simulink subsystem "rss_ECUCircuitry"  (R2024a)
settings: Solver=VariableStepAuto  StartTime=0.0  StopTime=10.0  RelTol=1e-3
libraries: fl_lib x41, nesl_utility x19, ee_lib x1
settings Model: Creator=pav2ofo  LastModifiedBy=pav2ofo

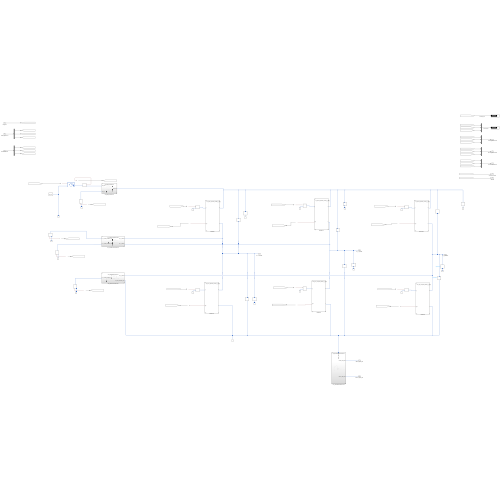
[thumbnail: Simulink's stored preview of the top-level diagram]
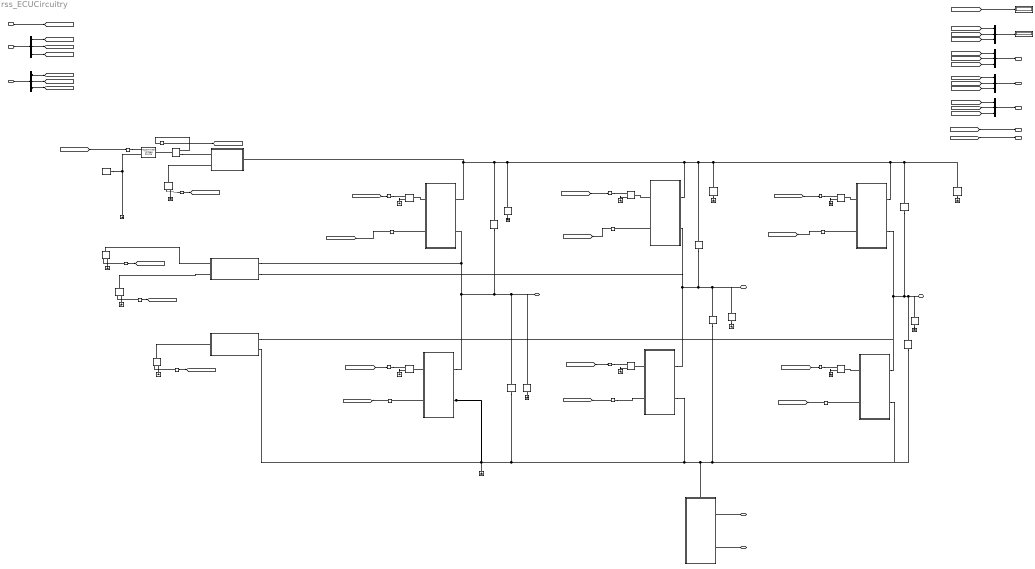
== system rss_ECUCircuitry ==
  vtSplyVolt : Inport
  iXYZHighGateCurr : Inport  Port=2
  iXYZLowGateCurr : Inport  Port=3
  Capacitor1 : fl_lib/Electrical/Electrical Elements/Capacitor  c=cstDrnPhsCpct F  r=cstDrnPhsCpcrRstn Ohm  g=0 1/Ohm  i_specify=off  i_priority=None  i=0 A  i_nominal_specify=off  i_nominal_value=1  i_nominal_unit=A  v_specify=off  v_priority=None  v=0 V  v_nominal_specify=off  v_nominal_value=1  v_nominal_unit=V  vc_specify=off  vc_priority=High  vc=0 V  vc_nominal_specify=off  vc_nominal_value=1  vc_nominal_unit=V
  Capacitor10 : fl_lib/Electrical/Electrical Elements/Capacitor  c=cstPhsGrndCpct F  r=cstPhsGrndCpcrRstn Ohm  g=0 1/Ohm  i_specify=off  i_priority=None  i=0 A  i_nominal_specify=off  i_nominal_value=1  i_nominal_unit=A  v_specify=off  v_priority=None  v=0 V  v_nominal_specify=off  v_nominal_value=1  v_nominal_unit=V  vc_specify=off  vc_priority=High  vc=0 V  vc_nominal_specify=off  vc_nominal_value=1  vc_nominal_unit=V
  Capacitor11 : fl_lib/Electrical/Electrical Elements/Capacitor  c=cstPhsGrndCpct F  r=cstPhsGrndCpcrRstn Ohm  g=0 1/Ohm  i_specify=off  i_priority=None  i=0 A  i_nominal_specify=off  i_nominal_value=1  i_nominal_unit=A  v_specify=off  v_priority=None  v=0 V  v_nominal_specify=off  v_nominal_value=1  v_nominal_unit=V  vc_specify=off  vc_priority=High  vc=0 V  vc_nominal_specify=off  vc_nominal_value=1  vc_nominal_unit=V
  Capacitor12 : fl_lib/Electrical/Electrical Elements/Capacitor  c=cstPhsSrcCpct F  r=cstPhsSrcCpcrRstn Ohm  g=0 1/Ohm  i_specify=off  i_priority=None  i=0 A  i_nominal_specify=off  i_nominal_value=1  i_nominal_unit=A  v_specify=off  v_priority=None  v=0 V  v_nominal_specify=off  v_nominal_value=1  v_nominal_unit=V  vc_specify=off  vc_priority=High  vc=0 V  vc_nominal_specify=off  vc_nominal_value=1  vc_nominal_unit=V
  Capacitor2 : fl_lib/Electrical/Electrical Elements/Capacitor  c=cstDrnPhsCpct F  r=cstDrnPhsCpcrRstn Ohm  g=0 1/Ohm  i_specify=off  i_priority=None  i=0 A  i_nominal_specify=off  i_nominal_value=1  i_nominal_unit=A  v_specify=off  v_priority=None  v=0 V  v_nominal_specify=off  v_nominal_value=1  v_nominal_unit=V  vc_specify=off  vc_priority=High  vc=0 V  vc_nominal_specify=off  vc_nominal_value=1  vc_nominal_unit=V
  Capacitor3 : fl_lib/Electrical/Electrical Elements/Capacitor  c=cstDrnGrndCpct F  r=cstDrnGrndCpcrRstn Ohm  g=0 1/Ohm  i_specify=off  i_priority=None  i=0 A  i_nominal_specify=off  i_nominal_value=1  i_nominal_unit=A  v_specify=off  v_priority=None  v=0 V  v_nominal_specify=off  v_nominal_value=1  v_nominal_unit=V  vc_specify=off  vc_priority=High  vc=0 V  vc_nominal_specify=off  vc_nominal_value=1  vc_nominal_unit=V
  Capacitor4 : fl_lib/Electrical/Electrical Elements/Capacitor  c=cstDrnGrndCpct F  r=cstDrnGrndCpcrRstn Ohm  g=0 1/Ohm  i_specify=off  i_priority=None  i=0 A  i_nominal_specify=off  i_nominal_value=1  i_nominal_unit=A  v_specify=off  v_priority=None  v=0 V  v_nominal_specify=off  v_nominal_value=1  v_nominal_unit=V  vc_specify=off  vc_priority=High  vc=0 V  vc_nominal_specify=off  vc_nominal_value=1  vc_nominal_unit=V
  Capacitor5 : fl_lib/Electrical/Electrical Elements/Capacitor  c=cstDrnPhsCpct F  r=cstDrnPhsCpcrRstn Ohm  g=0 1/Ohm  i_specify=off  i_priority=None  i=0 A  i_nominal_specify=off  i_nominal_value=1  i_nominal_unit=A  v_specify=off  v_priority=None  v=0 V  v_nominal_specify=off  v_nominal_value=1  v_nominal_unit=V  vc_specify=off  vc_priority=High  vc=0 V  vc_nominal_specify=off  vc_nominal_value=1  vc_nominal_unit=V
  Capacitor6 : fl_lib/Electrical/Electrical Elements/Capacitor  c=cstDrnGrndCpct F  r=cstDrnGrndCpcrRstn Ohm  g=0 1/Ohm  i_specify=off  i_priority=None  i=0 A  i_nominal_specify=off  i_nominal_value=1  i_nominal_unit=A  v_specify=off  v_priority=None  v=0 V  v_nominal_specify=off  v_nominal_value=1  v_nominal_unit=V  vc_specify=off  vc_priority=High  vc=0 V  vc_nominal_specify=off  vc_nominal_value=1  vc_nominal_unit=V
  Capacitor7 : fl_lib/Electrical/Electrical Elements/Capacitor  c=cstPhsSrcCpct F  r=cstPhsSrcCpcrRstn Ohm  g=0 1/Ohm  i_specify=off  i_priority=None  i=0 A  i_nominal_specify=off  i_nominal_value=1  i_nominal_unit=A  v_specify=off  v_priority=None  v=0 V  v_nominal_specify=off  v_nominal_value=1  v_nominal_unit=V  vc_specify=off  vc_priority=High  vc=0 V  vc_nominal_specify=off  vc_nominal_value=1  vc_nominal_unit=V
  Capacitor8 : fl_lib/Electrical/Electrical Elements/Capacitor  c=cstPhsGrndCpct F  r=cstPhsGrndCpcrRstn Ohm  g=0 1/Ohm  i_specify=off  i_priority=None  i=0 A  i_nominal_specify=off  i_nominal_value=1  i_nominal_unit=A  v_specify=off  v_priority=None  v=0 V  v_nominal_specify=off  v_nominal_value=1  v_nominal_unit=V  vc_specify=off  vc_priority=High  vc=0 V  vc_nominal_specify=off  vc_nominal_value=1  vc_nominal_unit=V
  Capacitor9 : fl_lib/Electrical/Electrical Elements/Capacitor  c=cstPhsSrcCpct F  r=cstPhsSrcCpcrRstn Ohm  g=0 1/Ohm  i_specify=off  i_priority=None  i=0 A  i_nominal_specify=off  i_nominal_value=1  i_nominal_unit=A  v_specify=off  v_priority=None  v=0 V  v_nominal_specify=off  v_nominal_value=1  v_nominal_unit=V  vc_specify=off  vc_priority=High  vc=0 V  vc_nominal_specify=off  vc_nominal_value=1  vc_nominal_unit=V
  Controlled Current Source{7..12} (6 alike) : fl_lib/Electrical/Electrical Sources/Controlled Current Source
  Current Sensor : fl_lib/Electrical/Electrical Sensors/Current Sensor
  Demux : Demux  Outputs=3
  Demux1 : Demux  Outputs=3
  Display : Display
  Display1 : Display
  Electrical Reference{,1,3..7,13..14,16..24} (18 alike) : fl_lib/Electrical/Electrical Elements/Electrical Reference
  MOSFET{1..6} (6 alike) : Subsystem  ReferencedSubsystem=rss_spice_imported_mosfet_p_gate_charge_circuit
  Mux{1..4} (4 alike) : Mux  Inputs=3
  PS-Simulink Converter{,14..15,20,23,25..30} (11 alike) : nesl_utility/PS-Simulink Converter  PhysicalDomain=network_engine_domain  SubClassName=ps_output  LeftPortType=input  RightPortType=output  PseudoPeriodic=off  Frequencies=[]  VectorFormat=inherit  Unit=inherit  AffineConversion=off
  Programmable Voltage Source8 : ee_lib/Sources/Programmable Voltage Source  magnitude_type=ee.enum.timechanging.constant  ac_magnitude=0 V  magn_ramp=1 V/s  magn_step=1 V  magn_modu_magn=1 V  magn_modu_freq=1 Hz  magn_t1=1 s  magn_t2=2 s  frequency_type=ee.enum.timechanging.constant  ac_frequency=60 Hz  freq_ramp=1 Hz/s  freq_step=1 Hz  freq_modu_magn=1 Hz  freq_modu_freq=1 Hz  freq_t1=1 s  freq_t2=2 s  phase_type=ee.enum.timechanging.constant  ac_shift=0 deg  phase_ramp=1 deg/s  phase_step=1 deg  phase_modu_magn=1 deg  phase_modu_freq=1 Hz  phase_t1=1 s  phase_t2=2 s  dc_type=ee.enum.timechanging.external  dc_voltage=0 V  dc_ramp=1 V/s  dc_step=1 V  dc_modu_magn=1 V  dc_modu_freq=1 Hz  dc_t1=1 s  dc_t2=2 s  harmonic_option=0  harmonic_orders=[5, 7, 11, 13]  harmonic_ratios=[.1, .1, .1, .1]  harmonic_shifts=[0, 0, 0, 0] deg  harmonic_t1=-inf s  harmonic_t2=inf s  noise_mode=0  PSD=0 V^2/Hz  repeatability=1  auto_seed=0  user_seed=0  sample_time=1e-3 s  i_specify=off  i_priority=None  i=0 A  i_nominal_specify=off  i_nominal_value=1  i_nominal_unit=A  v_specify=off  v_priority=None  v=0 V  v_nominal_specify=off  v_nominal_value=1  v_nominal_unit=V
      settings: InternalSimscapePortConfiguration="{\"Bottom\":[],\"Left\":[{\"id\":\"p\",\"label\":\"+\",\"type\":\"foundation.electrical.electrical\"}],\"Right\":[{\"id\":\"ext_dc\",\"label\":\"DC\",\"type\":\"input\"},{\"id\":\"n\",\"label\":\"-\",\"type\":\"foundation.electrical.electrical\"}],\"Top\":[]}"
  Simulink-PS Converter{7..13} (7 alike) : nesl_utility/Simulink-PS Converter  PhysicalDomain=network_engine_domain  SubClassName=ps_input  LeftPortType=input  RightPortType=output  PseudoPeriodic=off  Frequencies=[]  NoiseDistribution=none  NoiseParameters=[]  Unit=1  AffineConversion=off  FilteringAndDerivatives=zero  SimscapeFilterOrder=1  InputFilterTimeConstant=0.001  UdotUserProvided=0
  Solver Configuration1 : nesl_utility/Solver Configuration  PhysicalDomain=network_engine_domain  SubClassName=solver  LeftPortType=input  RightPortType=generic  Tones=[]  Harmonics=[]  SimulateNoise=off  Profile=off  UseLocalSampling=off  EnableSwitchedLinearOptims=on  FrequencyDomain=off  UseCCode=off  RelTol=0.001  AbsTol=0.001  MinStep=1e-09  ToWorkspace=off  RevertToSquareIcSolve=off  NumHomotopyIterations=100  PhasorMode=off  PhasorModeNumHarmonics=1  ConsistencySolver=NEWTON_XTOL_AFTER_FTOL  IndexReductionMethod=None  DoDC=off  ResidualTolerance=1e-09  ConsistencyTolSource=GLOBAL  ConsistencyAbsTol=0.001  ConsistencyRelTol=0.001  ConsistencyTolFactor=1e-2  UseLocalSolver=on  LocalSolverChoice=NE_BACKWARD_EULER_ADVANCER  ResolveIndetEquations=off  FunctionEvalNumThread=1  LocalSolverSampleTime=cstSpicInvtMdlSampTime  DoFixedCost=on  MaxNonlinIter=3  MaxModeIter=2  ComputeImpulses=off  ImpulseIterations=2  LinearAlgebra=auto  LinearAlgebraNumThread=0  EquationFormulation=NE_TIME_EF  DelaysMemoryBudget=1024  AutomaticFiltering=off  FilteringTimeConstant=0.001  PartitionStorageMethod=AS_NEEDED  PartitionMemoryBudget=1024  PartitionMethod=ROBUST  MultibodyUseLocalSolver=off  MultibodyLocalSolverChoice=ODE1  MultibodyLocalSolverSampleTime=0.001
  Voltage Sensor{7,9,13,16} (4 alike) : fl_lib/Electrical/Electrical Sensors/Voltage Sensor
  rss_BatteryFilterCircuit : Subsystem  ReferencedSubsystem=rss_BatteryFilterCircuit
      settings: PortSchema="{\"entries\":[{\"content\":{\"sides\":[{\"content\":{},\"type\":\"ConnectorPlacement.EquallySpacedRectSide\",\"uuid\":\"af59638e-9135-4340-92f0-20c1fae13fbc\"},{\"content\":{\"side\":\"RIGHT\"},\"type\":\"ConnectorPlacement.EquallySpacedRectSide\",\"uuid\":\"9dd79a46-d4bd-4a1f-9771-2bd83095d194\"},{\"content\":{\"connectorIds\":[\"LConn1\"],\"side\":\"TOP\"},\"type\":\"ConnectorPlacement.EquallySpacedRectSide\",\"uuid\":\"2425462a-e1fd-4da5-99fb-ecd6b870d2ba\"},{\"content\":{\"connectorIds\":[\"RConn1\",\"LConn2\"],\"side\":\"BOTTOM\"},\"type\":\"ConnectorPlacement.EquallySpacedRectSide\",\"uuid\":\"7f50a858-c489-43c1-aa02-240ba8096b11\"}]},\"type\":\"ConnectorPlacement.EquallySpacedConnector\",\"uuid\":\"7f481854-5cd2-45e2-9053-749c0d657114\"}],\"packageUris\":[\"http://schema.mathworks.com/mf0/Connector/R2020b\"],\"version\":\"1.0\"}"
  sss_ShuntMeasrementCircuit : Subsystem  ReferencedSubsystem=rss_ShuntMeasurementCircuit
      settings: PortSchema="{\"entries\":[{\"content\":{\"sides\":[{\"content\":{},\"type\":\"ConnectorPlacement.EquallySpacedRectSide\",\"uuid\":\"41c7778a-6430-4999-a854-4734d5e300a5\"},{\"content\":{\"connectorIds\":[\"RConn1\",\"RConn2\"],\"side\":\"RIGHT\"},\"type\":\"ConnectorPlacement.EquallySpacedRectSide\",\"uuid\":\"34b88b4c-3327-4ed5-9a31-d44316fa4d1d\"},{\"content\":{\"connectorIds\":[\"LConn1\"],\"side\":\"TOP\"},\"type\":\"ConnectorPlacement.EquallySpacedRectSide\",\"uuid\":\"2367d310-acba-4c49-b790-8e354dd0d98f\"}]},\"type\":\"ConnectorPlacement.EquallySpacedConnector\",\"uuid\":\"fb95dde9-175f-463b-81f5-aa4ba5041aeb\"}],\"packageUris\":[\"http://schema.mathworks.com/mf0/Connector/R2020b\"],\"version\":\"1.0\"}"
  sss_XYPhaseTerminalCircuit : Subsystem  ReferencedSubsystem=rss_XYPhaseTerminalCircuit
      settings: PortSchema="{\"entries\":[{\"content\":{\"sides\":[{\"content\":{\"connectorIds\":[\"RConn3\",\"RConn4\"]},\"type\":\"ConnectorPlacement.EquallySpacedRectSide\",\"uuid\":\"a1d92818-0d9b-4f85-8c09-17a27c8f3dda\"},{\"content\":{\"connectorIds\":[\"RConn1\",\"RConn2\"],\"side\":\"RIGHT\"},\"type\":\"ConnectorPlacement.EquallySpacedRectSide\",\"uuid\":\"4fd32171-b09b-4594-8c71-47bfb70041de\"},{\"content\":{\"side\":\"TOP\"},\"type\":\"ConnectorPlacement.EquallySpacedRectSide\",\"uuid\":\"447e300e-4af2-4486-95f9-9bf74e26982a\"}]},\"type\":\"ConnectorPlacement.EquallySpacedConnector\",\"uuid\":\"7b10fa05-4116-4e12-9084-742caf78674f\"}],\"packageUris\":[\"http://schema.mathworks.com/mf0/Connector/R2020b\"],\"version\":\"1.0\"}"
  sss_ZPhaseTerminalCircuit : Subsystem  ReferencedSubsystem=rss_ZPhaseTerminalCircuit
      settings: PortSchema="{\"entries\":[{\"content\":{\"sides\":[{\"content\":{\"connectorIds\":[\"RConn2\"]},\"type\":\"ConnectorPlacement.EquallySpacedRectSide\",\"uuid\":\"9795e9b2-2c73-4919-87b4-9a5ec4887685\"},{\"content\":{\"connectorIds\":[\"RConn1\",\"RConn3\"],\"side\":\"RIGHT\"},\"type\":\"ConnectorPlacement.EquallySpacedRectSide\",\"uuid\":\"1f799a50-fc66-4f81-99b2-70dc99e72627\"},{\"content\":{\"side\":\"TOP\"},\"type\":\"ConnectorPlacement.EquallySpacedRectSide\",\"uuid\":\"0eea85e6-56d4-400e-93a3-18ac9e3a1609\"}]},\"type\":\"ConnectorPlacement.EquallySpacedConnector\",\"uuid\":\"ce5e4492-8dc3-44ce-aa1e-b210db680c4d\"}],\"packageUris\":[\"http://schema.mathworks.com/mf0/Connector/R2020b\"],\"version\":\"1.0\"}"
  EL_X_PHASE : PMIOPort  Side=Right
  EL_Y_PHASE : PMIOPort  Port=2  Side=Right
  EL_Z_PHASE : PMIOPort  Port=3  Side=Right
  SHUNT_POS_PIN : PMIOPort  Port=4  Side=Right
  SHUNT_NEG_PIN : PMIOPort  Port=5  Side=Right
  vtXYZHighGateSrcVolt : Outport
  vtXYZHighSrcGrndVolt : Outport  Port=2
  vtXYZLowGateSrcVolt : Outport  Port=3
  vtLowSrcGrndVolt : Outport  Port=4
  vtDHVolt : Outport  Port=5
  wires:
  Demux/3 -> [iZLowGateCurr]
  [vtYLowGateSrcVolt] -> Mux4/2
  [vtYHighSrcGrndVolt] -> Mux3/2
  [vtZLineVolt] -> Mux2/3
  [vtYLineVolt] -> Mux2/2
  PS-Simulink Converter30/1 -> [vtZLowGateSrcVolt]
  Mux1/1 -> vtXYZHighGateSrcVolt/1
  Mux4/1 -> vtXYZLowGateSrcVolt/1
  [vtDHVolt] -> vtDHVolt/1
  [vtZLowGateSrcVolt] -> Mux4/3
  iXYZLowGateCurr/1 -> Demux/1
  Demux1/1 -> [iXHighGateCurr]
  [vtYHighGateSrcVolt] -> Mux1/2
  PS-Simulink Converter25/1 -> [vtXHighGateSrcVolt]
  PS-Simulink Converter29/1 -> [vtZHighGateSrcVolt]
  [iZHighGateCurr] -> Simulink-PS Converter12/1
  PS-Simulink Converter28/1 -> [vtYLowGateSrcVolt]
  [vtXHighGateSrcVolt] -> Mux1/1
  PS-Simulink Converter26/1 -> [vtXLowGateSrcVolt]
  iXYZHighGateCurr/1 -> Demux1/1
  [iMeasSplyCurr] -> Display/1  "iMeasSplyCurr"
  [iXLowGateCurr] -> Simulink-PS Converter9/1
  Mux2/1 -> Display1/1  "vtXYZLineVolt"
  PS-Simulink Converter27/1 -> [vtYHighGateSrcVolt]
  [vtXLineVolt] -> Mux2/1
  [iXHighGateCurr] -> Simulink-PS Converter7/1
  Demux/2 -> [iYLowGateCurr]
  [vtZHighSrcGrndVolt] -> Mux3/3
  Demux1/3 -> [iZHighGateCurr]
  [iZLowGateCurr] -> Simulink-PS Converter13/1
  vtSplyVolt/1 -> [vtSplyVolt]
  [iYHighGateCurr] -> Simulink-PS Converter10/1
  Mux3/1 -> vtXYZHighSrcGrndVolt/1
  [vtZHighGateSrcVolt] -> Mux1/3
  [vtLowSrcGrndVolt] -> vtLowSrcGrndVolt/1
  [iYLowGateCurr] -> Simulink-PS Converter11/1
  Demux/1 -> [iXLowGateCurr]
  Demux1/2 -> [iYHighGateCurr]
  [vtXLowGateSrcVolt] -> Mux4/1
  [vtXHighSrcGrndVolt] -> Mux3/1
  PS-Simulink Converter/1 -> [iMeasSplyCurr]
  PS-Simulink Converter14/1 -> [vtDHVolt]
  [vtSplyVolt] -> Simulink-PS Converter8/1
  PS-Simulink Converter23/1 -> [vtZHighSrcGrndVolt]
  PS-Simulink Converter20/1 -> [vtYHighSrcGrndVolt]
  PS-Simulink Converter15/1 -> [vtXHighSrcGrndVolt]
  connections:
  MOSFET2/RConn1 -- Capacitor8/LConn1 -- EL_X_PHASE/RConn1 -- Capacitor7/LConn1 -- Capacitor2/RConn1 -- sss_XYPhaseTerminalCircuit/RConn1 -- MOSFET1/RConn2
  Capacitor6/LConn1 -- MOSFET5/RConn1 -- Capacitor4/LConn1 -- Capacitor1/LConn1 -- Capacitor2/LConn1 -- rss_BatteryFilterCircuit/LConn1 -- MOSFET1/RConn1 -- Capacitor3/LConn1 -- MOSFET3/RConn1 -- Capacitor5/LConn1
  MOSFET2/RConn2 -- Capacitor7/RConn1 -- Capacitor12/RConn1 -- MOSFET6/RConn2 -- Capacitor9/RConn1 -- sss_ShuntMeasrementCircuit/LConn1 -- MOSFET4/RConn2 -- sss_ZPhaseTerminalCircuit/RConn3 -- Electrical Reference24/LConn1
  MOSFET4/RConn1 -- Capacitor10/LConn1 -- EL_Y_PHASE/RConn1 -- Capacitor9/LConn1 -- Capacitor1/RConn1 -- MOSFET3/RConn2 -- sss_XYPhaseTerminalCircuit/RConn2
  MOSFET5/RConn2 -- Capacitor11/LConn1 -- EL_Z_PHASE/RConn1 -- Capacitor12/LConn1 -- Capacitor5/RConn1 -- sss_ZPhaseTerminalCircuit/RConn1 -- MOSFET6/RConn1
  Electrical Reference/LConn1 -- Solver Configuration1/RConn1 -- Programmable Voltage Source8/RConn2
  Simulink-PS Converter11/RConn1 -- Controlled Current Source10/RConn1
  MOSFET1/LConn2 -- PS-Simulink Converter25/LConn1
  MOSFET2/LConn1 -- Controlled Current Source8/LConn1
  Electrical Reference21/LConn1 -- Controlled Current Source10/RConn2
  Simulink-PS Converter7/RConn1 -- Controlled Current Source7/RConn1
  MOSFET3/LConn2 -- PS-Simulink Converter27/LConn1
  Simulink-PS Converter10/RConn1 -- Controlled Current Source9/RConn1
  MOSFET4/LConn1 -- Controlled Current Source10/LConn1
  PS-Simulink Converter28/LConn1 -- MOSFET4/LConn2
  Electrical Reference20/LConn1 -- Controlled Current Source9/RConn2
  MOSFET6/LConn1 -- Controlled Current Source11/LConn1
  Simulink-PS Converter13/RConn1 -- Controlled Current Source11/RConn1
  MOSFET5/LConn1 -- Controlled Current Source12/LConn1
  MOSFET3/LConn1 -- Controlled Current Source9/LConn1
  Electrical Reference22/LConn1 -- Controlled Current Source12/RConn2
  Electrical Reference19/LConn1 -- Controlled Current Source8/RConn2
  MOSFET1/LConn1 -- Controlled Current Source7/LConn1
  MOSFET2/LConn2 -- PS-Simulink Converter26/LConn1
  Simulink-PS Converter9/RConn1 -- Controlled Current Source8/RConn1
  Electrical Reference23/LConn1 -- Controlled Current Source11/RConn2
  Simulink-PS Converter12/RConn1 -- Controlled Current Source12/RConn1
  MOSFET6/LConn2 -- PS-Simulink Converter30/LConn1
  Electrical Reference18/LConn1 -- Controlled Current Source7/RConn2
  MOSFET5/LConn2 -- PS-Simulink Converter29/LConn1
  Current Sensor/RConn2 -- rss_BatteryFilterCircuit/RConn1
  PS-Simulink Converter14/LConn1 -- Voltage Sensor7/RConn1
  PS-Simulink Converter/LConn1 -- Current Sensor/RConn1
  Simulink-PS Converter8/RConn1 -- Programmable Voltage Source8/RConn1
  Electrical Reference13/LConn1 -- Voltage Sensor7/RConn2
  Current Sensor/LConn1 -- Programmable Voltage Source8/LConn1
  Voltage Sensor7/LConn1 -- rss_BatteryFilterCircuit/LConn2
  SHUNT_POS_PIN/RConn1 -- sss_ShuntMeasrementCircuit/RConn1
  SHUNT_NEG_PIN/RConn1 -- sss_ShuntMeasrementCircuit/RConn2
  Electrical Reference17/LConn1 -- Voltage Sensor16/RConn2
  PS-Simulink Converter23/LConn1 -- Voltage Sensor16/RConn1
  Voltage Sensor16/LConn1 -- sss_ZPhaseTerminalCircuit/RConn2
  Electrical Reference16/LConn1 -- Voltage Sensor13/RConn2
  PS-Simulink Converter20/LConn1 -- Voltage Sensor13/RConn1
  Voltage Sensor13/LConn1 -- sss_XYPhaseTerminalCircuit/RConn4
  Electrical Reference14/LConn1 -- Voltage Sensor9/RConn2
  PS-Simulink Converter15/LConn1 -- Voltage Sensor9/RConn1
  Voltage Sensor9/LConn1 -- sss_XYPhaseTerminalCircuit/RConn3
  Capacitor6/RConn1 -- Electrical Reference4/LConn1
  Capacitor11/RConn1 -- Electrical Reference6/LConn1
  Capacitor4/RConn1 -- Electrical Reference3/LConn1
  Capacitor10/RConn1 -- Electrical Reference7/LConn1
  Electrical Reference1/LConn1 -- Capacitor3/RConn1
  Electrical Reference5/LConn1 -- Capacitor8/RConn1
